simulink subsystem "rss_SensAgCalibNeed"  (R2023a)
settings: Solver=VariableStepAuto  StartTime=0.0  StopTime=10.0  RelTol=1e-3
undefined symbols (not defined in the file): Cdbl_numCalibAlgnNum, Cdbl_trqTqMaxVal, ENM_SYS_STATUS, Gs16_trqRefTqAlgnVal_C, Gu16_ctAlgnAlPhStCnt_C, Gu16_ctAlgnBePhStCnt_C, Gu16_ctAlgnTmpFailStCnt_C, Gu16_ctAlgnWaitAlStCnt_C, Gu16_ctAlgnWaitBeStCnt_C, Gu16_phiAlgnAlPhElecAg_C, Gu16_phiAlgnBePhElecAg_C, Gu16_phiMinAlgnElecAngDvt_C, Gu16_phiTheoBePhElecAg_C
libraries: simulink x1, lib_configurable_parameter x1, vhit_control_library x1, lib_conversion x1
settings Model: Creator=YXQ1WX  LastModifiedBy=xiaoqiang.yuan
settings OptimizationCC: ReuseModelBlockBuffer=off

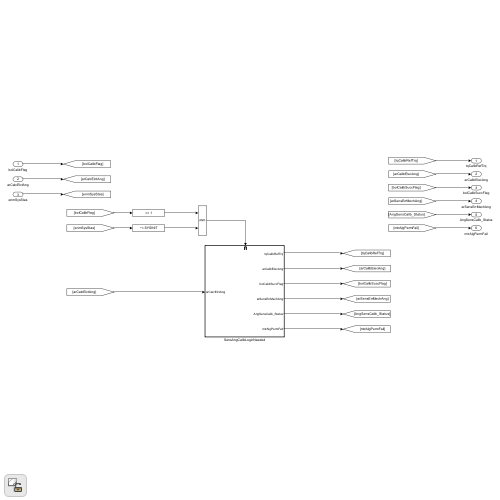
[thumbnail: Simulink's stored preview of the top-level diagram]
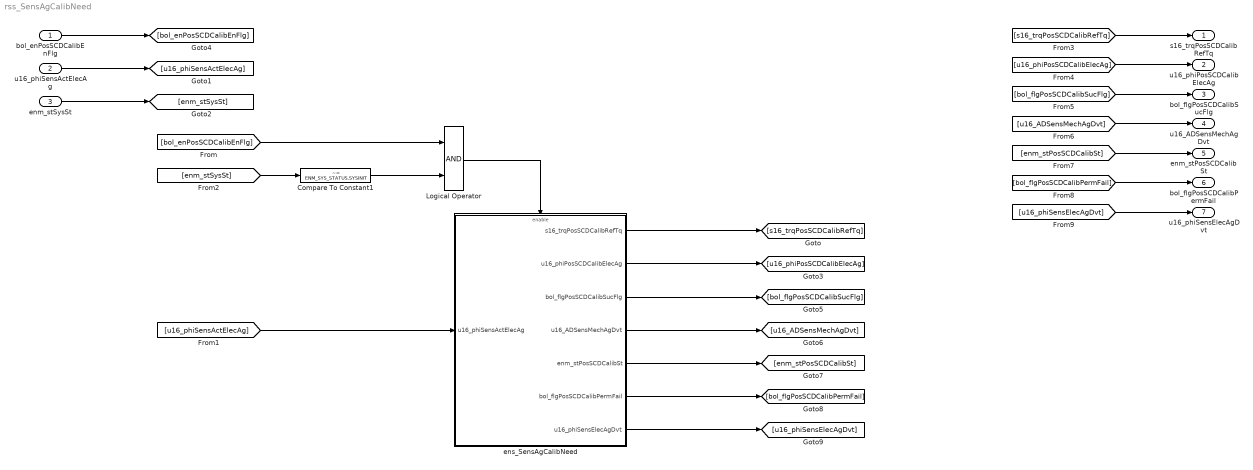
== system rss_SensAgCalibNeed ==
  bol_enPosSCDCalibEnFlg : Inport  OutDataTypeStr=boolean
  u16_phiSensActElecAg : Inport  Port=2  OutDataTypeStr=dt_RadAng_u16r15b0
  enm_stSysSt : Inport  Port=3  OutDataTypeStr=Enum: ENM_SYS_STATUS
  Compare To Constant1 : simulink/Logic and Bit Operations/Compare To Constant  relop=~=  const=ENM_SYS_STATUS.SYSINIT  OutDataTypeStr=boolean
  Logical Operator : Logic  AllPortsSameDT=off  OutDataTypeStr=boolean
  ens_SensAgCalibNeed : Subsystem
  s16_trqPosSCDCalibRefTq : Outport  OutDataTypeStr=dt_Standardize_s16p15b0
  u16_phiPosSCDCalibElecAg : Outport  Port=2  OutDataTypeStr=dt_RadAng_u16r15b0
  bol_flgPosSCDCalibSucFlg : Outport  Port=3  OutDataTypeStr=boolean
  u16_ADSensMechAgDvt : Outport  Port=4  OutDataTypeStr=uint16
  enm_stPosSCDCalibSt : Outport  Port=5  OutDataTypeStr=Enum: ENM_AG_SENS_CALIB_STATUS
  bol_flgPosSCDCalibPermFail : Outport  Port=6  OutDataTypeStr=boolean
  u16_phiSensElecAgDvt : Outport  Port=7  OutDataTypeStr=dt_RadAng_u16r15b0
  wires:
  [u16_phiSensActElecAg] -> ens_SensAgCalibNeed/1(u16_phiSensActElecAg)
  ens_SensAgCalibNeed/1(s16_trqPosSCDCalibRefTq) -> [s16_trqPosSCDCalibRefTq]
  ens_SensAgCalibNeed/2(u16_phiPosSCDCalibElecAg) -> [u16_phiPosSCDCalibElecAg]
  ens_SensAgCalibNeed/3(bol_flgPosSCDCalibSucFlg) -> [bol_flgPosSCDCalibSucFlg]
  ens_SensAgCalibNeed/4(u16_ADSensMechAgDvt) -> [u16_ADSensMechAgDvt]
  ens_SensAgCalibNeed/5(enm_stPosSCDCalibSt) -> [enm_stPosSCDCalibSt]
  ens_SensAgCalibNeed/6(bol_flgPosSCDCalibPermFail) -> [bol_flgPosSCDCalibPermFail]
  Compare To Constant1/1 -> Logical Operator/2
  Logical Operator/1 -> ens_SensAgCalibNeed/Enable
  [bol_enPosSCDCalibEnFlg] -> Logical Operator/1
  [enm_stSysSt] -> Compare To Constant1/1
  bol_enPosSCDCalibEnFlg/1 -> [bol_enPosSCDCalibEnFlg]
  u16_phiSensActElecAg/1 -> [u16_phiSensActElecAg]
  enm_stSysSt/1 -> [enm_stSysSt]
  [s16_trqPosSCDCalibRefTq] -> s16_trqPosSCDCalibRefTq/1
  [u16_phiPosSCDCalibElecAg] -> u16_phiPosSCDCalibElecAg/1
  [bol_flgPosSCDCalibSucFlg] -> bol_flgPosSCDCalibSucFlg/1
  [u16_ADSensMechAgDvt] -> u16_ADSensMechAgDvt/1
  [enm_stPosSCDCalibSt] -> enm_stPosSCDCalibSt/1
  [bol_flgPosSCDCalibPermFail] -> bol_flgPosSCDCalibPermFail/1
  [u16_phiSensElecAgDvt] -> u16_phiSensElecAgDvt/1
  ens_SensAgCalibNeed/7(u16_phiSensElecAgDvt) -> [u16_phiSensElecAgDvt]

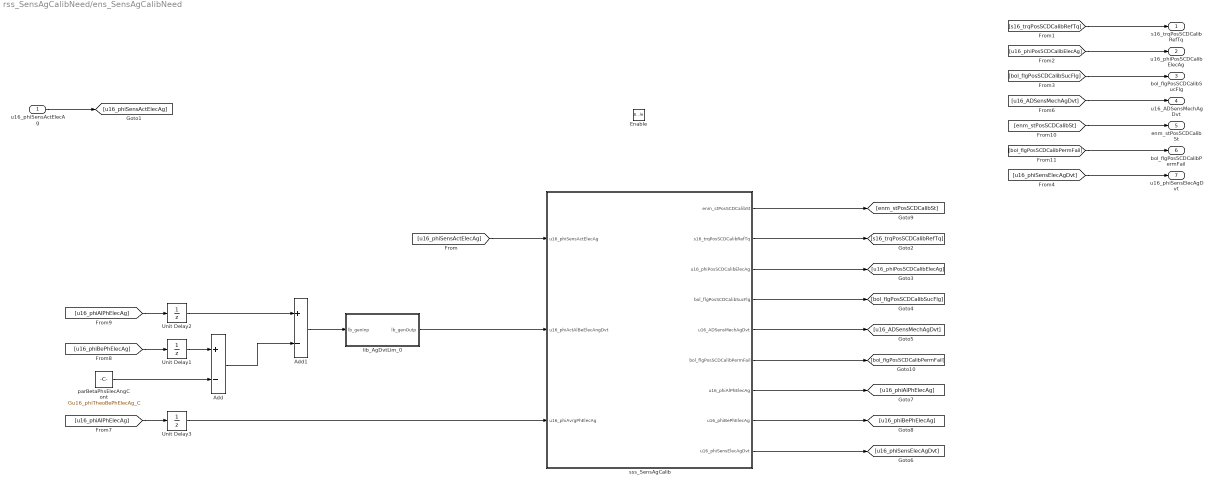
== system rss_SensAgCalibNeed/ens_SensAgCalibNeed ==
  u16_phiSensActElecAg : Inport
  Enable : EnablePort
  Add : Sum  Inputs=+-  RndMeth=Simplest  OutDataTypeStr=Inherit: Same as first input
  Add1 : Sum  Inputs=+-  RndMeth=Simplest  OutDataTypeStr=Inherit: Same as first input
  Unit Delay1 : UnitDelay  SampleTime=-1  HasFrameUpgradeWarning=on
  Unit Delay2 : UnitDelay  SampleTime=-1  HasFrameUpgradeWarning=on
  Unit Delay3 : UnitDelay  SampleTime=-1  HasFrameUpgradeWarning=on
  lib_AgDvtLim_0 : Subsystem
  parBetaPhsElecAngCont : Constant  Value=Gu16_phiTheoBePhElecAg_C
  sss_SensAgCalib : Subsystem
  s16_trqPosSCDCalibRefTq : Outport
  u16_phiPosSCDCalibElecAg : Outport  Port=2
  bol_flgPosSCDCalibSucFlg : Outport  Port=3
  u16_ADSensMechAgDvt : Outport  Port=4
  enm_stPosSCDCalibSt : Outport  Port=5
  bol_flgPosSCDCalibPermFail : Outport  Port=6
  u16_phiSensElecAgDvt : Outport  Port=7
  wires:
  [u16_phiSensElecAgDvt] -> u16_phiSensElecAgDvt/1
  sss_SensAgCalib/9(u16_phiSensElecAgDvt) -> [u16_phiSensElecAgDvt]
  [bol_flgPosSCDCalibPermFail] -> bol_flgPosSCDCalibPermFail/1
  parBetaPhsElecAngCont/1 -> Add/2
  lib_AgDvtLim_0/1(lb_genOutp) -> sss_SensAgCalib/2(u16_phiActAlBeElecAngDvt)
  Add1/1 -> lib_AgDvtLim_0/1(lb_genInp)
  Unit Delay3/1 -> sss_SensAgCalib/3(u16_phiAvrgPhElecAg)
  Unit Delay1/1 -> Add/1
  Add/1 -> Add1/2
  sss_SensAgCalib/6(bol_flgPosSCDCalibPermFail) -> [bol_flgPosSCDCalibPermFail]
  sss_SensAgCalib/3(u16_phiPosSCDCalibElecAg) -> [u16_phiPosSCDCalibElecAg]
  sss_SensAgCalib/5(u16_ADSensMechAgDvt) -> [u16_ADSensMechAgDvt]
  sss_SensAgCalib/7(u16_phiAlPhElecAg) -> [u16_phiAlPhElecAg]
  sss_SensAgCalib/8(u16_phiBePhElecAg) -> [u16_phiBePhElecAg]
  sss_SensAgCalib/4(bol_flgPosSCDCalibSucFlg) -> [bol_flgPosSCDCalibSucFlg]
  [u16_phiAlPhElecAg] -> Unit Delay3/1
  sss_SensAgCalib/2(s16_trqPosSCDCalibRefTq) -> [s16_trqPosSCDCalibRefTq]
  [bol_flgPosSCDCalibSucFlg] -> bol_flgPosSCDCalibSucFlg/1
  [u16_ADSensMechAgDvt] -> u16_ADSensMechAgDvt/1
  [u16_phiSensActElecAg] -> sss_SensAgCalib/1(u16_phiSensActElecAg)
  [s16_trqPosSCDCalibRefTq] -> s16_trqPosSCDCalibRefTq/1
  [u16_phiAlPhElecAg] -> Unit Delay2/1
  [u16_phiPosSCDCalibElecAg] -> u16_phiPosSCDCalibElecAg/1
  Unit Delay2/1 -> Add1/1
  [u16_phiBePhElecAg] -> Unit Delay1/1
  u16_phiSensActElecAg/1 -> [u16_phiSensActElecAg]
  [enm_stPosSCDCalibSt] -> enm_stPosSCDCalibSt/1
  sss_SensAgCalib/1(enm_stPosSCDCalibSt) -> [enm_stPosSCDCalibSt]

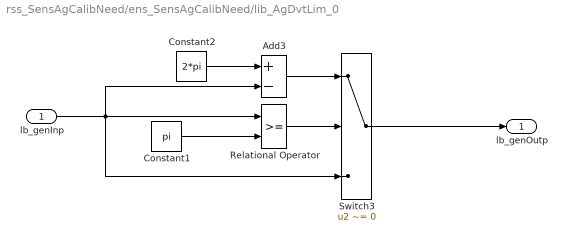
== system rss_SensAgCalibNeed/ens_SensAgCalibNeed/lib_AgDvtLim_0 ==
  lb_genInp : Inport
  Add3 : Sum  Inputs=+-  RndMeth=Simplest  OutDataTypeStr=Inherit: Same as first input
  Constant1 : Constant  Value=pi  OutDataTypeStr=dt_RadAng_u16r15b0
  Constant2 : Constant  Value=2*pi  OutDataTypeStr=dt_RadAng_u16r15b0
  Relational Operator : RelationalOperator  OutDataTypeStr=boolean  RndMeth=Simplest  InputSameDT=off
  Switch3 : Switch  Criteria=u2 ~= 0  RndMeth=Simplest  SaturateOnIntegerOverflow=off  InputSameDT=off  OutDataTypeStr=Inherit: Same as first input
  lb_genOutp : Outport
  wires:
  Relational Operator/1 -> Switch3/2
  Constant2/1 -> Add3/1
  Add3/1 -> Switch3/1
  lb_genInp/1 -> Relational Operator/1, Switch3/3, Add3/2
  Constant1/1 -> Relational Operator/2
  Switch3/1 -> lb_genOutp/1

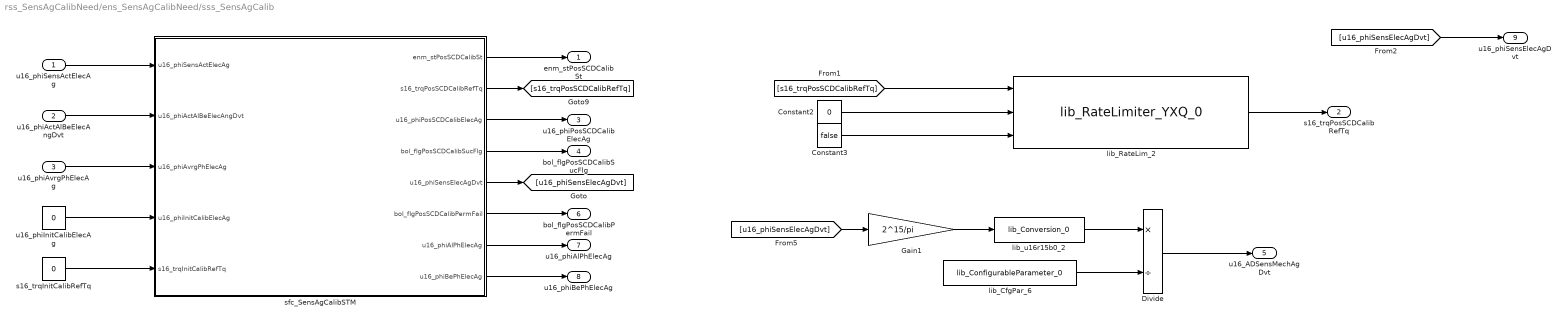
== system rss_SensAgCalibNeed/ens_SensAgCalibNeed/sss_SensAgCalib ==
  u16_phiSensActElecAg : Inport
  u16_phiActAlBeElecAngDvt : Inport  Port=2
  u16_phiAvrgPhElecAg : Inport  Port=3
  Constant2 : Constant  Value=0  OutDataTypeStr=dt_Standardize_s16p15b0
  Constant3 : Constant  Value=false  OutDataTypeStr=boolean
  Divide : Product  Inputs=*/  RndMeth=Simplest  OutDataTypeStr=Inherit: Same as first input
  Gain1 : Gain  Gain=2^15/pi  OutDataTypeStr=Inherit: Inherit via back propagation  RndMeth=Simplest
  lib_CfgPar_6 : lib_configurable_parameter/lib_ConfigurableParameter_0  lb_parCnfgPar=Gu8_numPPNum_C  lb_parDataType=Inherit: Inherit from 'Constant value'  lb_parUpLim=Cdbl_numPPNumMaxVal  lb_parLowLim=Cdbl_numPPNumMinVal
  lib_RateLim_2 : vhit_control_library/lib_RateLimiter_YXQ_0  lb_parSampTime=Cdbl_tiSlwTaskSmpTi  lb_parRiseSlewRate=Gs16_facAlgnTqRiseRate_C  lb_parFallSlewRate=Gs16_facAlgnTqFallRate_C  lb_parMaxInpVal=Cdbl_trqTqMaxVal  lb_parMinInpVal=-Cdbl_trqTqMaxVal
      settings: LibrarySourceBlock=lib_rate_limiter/lib_RateLimiter_0
  lib_u16r15b0_2 : lib_conversion/lib_Conversion_0  lb_parDataType=uint16  lb_parOutpMaxVal=[]  lb_parOutpMinVal=[]  lb_parSatFlag=off
  s16_trqInitCalibRefTq : Constant  Value=0  OutDataTypeStr=dt_Standardize_s16p15b0
  sfc_SensAgCalibSTM : Stateflow chart  TreatAsAtomicUnit=on
  u16_phiInitCalibElecAg : Constant  Value=0  OutDataTypeStr=dt_RadAng_u16r15b0
  enm_stPosSCDCalibSt : Outport
  s16_trqPosSCDCalibRefTq : Outport  Port=2
  u16_phiPosSCDCalibElecAg : Outport  Port=3
  bol_flgPosSCDCalibSucFlg : Outport  Port=4
  u16_ADSensMechAgDvt : Outport  Port=5
  bol_flgPosSCDCalibPermFail : Outport  Port=6
  u16_phiAlPhElecAg : Outport  Port=7
  u16_phiBePhElecAg : Outport  Port=8
  u16_phiSensElecAgDvt : Outport  Port=9
  wires:
  [u16_phiSensElecAgDvt] -> u16_phiSensElecAgDvt/1
  s16_trqInitCalibRefTq/1 -> sfc_SensAgCalibSTM/5(s16_trqInitCalibRefTq)
  u16_phiInitCalibElecAg/1 -> sfc_SensAgCalibSTM/4(u16_phiInitCalibElecAg)
  Constant3/1 -> lib_RateLim_2/3
  [s16_trqPosSCDCalibRefTq] -> lib_RateLim_2/1
  Constant2/1 -> lib_RateLim_2/2
  lib_RateLim_2/1 -> s16_trqPosSCDCalibRefTq/1
  Gain1/1 -> lib_u16r15b0_2/1
  lib_CfgPar_6/1 -> Divide/2
  Divide/1 -> u16_ADSensMechAgDvt/1
  [u16_phiSensElecAgDvt] -> Gain1/1
  lib_u16r15b0_2/1 -> Divide/1
  sfc_SensAgCalibSTM/3(u16_phiPosSCDCalibElecAg) -> u16_phiPosSCDCalibElecAg/1
  sfc_SensAgCalibSTM/2(s16_trqPosSCDCalibRefTq) -> [s16_trqPosSCDCalibRefTq]
  u16_phiActAlBeElecAngDvt/1 -> sfc_SensAgCalibSTM/2(u16_phiActAlBeElecAngDvt)
  u16_phiAvrgPhElecAg/1 -> sfc_SensAgCalibSTM/3(u16_phiAvrgPhElecAg)
  sfc_SensAgCalibSTM/8(u16_phiBePhElecAg) -> u16_phiBePhElecAg/1
  sfc_SensAgCalibSTM/7(u16_phiAlPhElecAg) -> u16_phiAlPhElecAg/1
  sfc_SensAgCalibSTM/5(u16_phiSensElecAgDvt) -> [u16_phiSensElecAgDvt]
  u16_phiSensActElecAg/1 -> sfc_SensAgCalibSTM/1(u16_phiSensActElecAg)
  sfc_SensAgCalibSTM/4(bol_flgPosSCDCalibSucFlg) -> bol_flgPosSCDCalibSucFlg/1
  sfc_SensAgCalibSTM/6(bol_flgPosSCDCalibPermFail) -> bol_flgPosSCDCalibPermFail/1
  sfc_SensAgCalibSTM/1(enm_stPosSCDCalibSt) -> enm_stPosSCDCalibSt/1

== stateflow chart rss_SensAgCalibNeed/ens_SensAgCalibNeed/sss_SensAgCalib/sfc_SensAgCalibSTM ==
  state ALIGN_ALPHA_PHASE1
    en:
    enm_stPosSCDCalibSt = ENM_AG_SENS_CALIB_STATUS.ALPHA_PHASE1;
    s16_trqPosSCDCalibRefTq = Gs16_trqRefTqAlgnVal_C;
    u16_phiPosSCDCalibElecAg = Gu16_phiAlgnAlPhElecAg_C;
    bol_flgPosSCDCalibSucFlg = false;
    bol_flgPosSCDCalibPermFail = false;
    u16_ctCalibStWaitCnt = uint16(0);
    du:
    u16_ctCalibStWaitCnt = u16_ctCalibStWaitCnt + uint16(1);
    ex:
    u16_ctCalibStWaitCnt = uint16(0);
    u16_phiAlPhElecAg = u16_phiSensActElecAg;
  state WAIT_ALPHA1
    en:
    enm_stPosSCDCalibSt = ENM_AG_SENS_CALIB_STATUS.WAIT_ALPHA1;
    s16_trqPosSCDCalibRefTq =s16_trqInitCalibRefTq;
    u16_phiPosSCDCalibElecAg = u16_phiInitCalibElecAg;
    bol_flgPosSCDCalibSucFlg = false;
    bol_flgPosSCDCalibPermFail = false;
    u16_ctCalibStWaitCnt = uint16(0);
    du:
    u16_ctCalibStWaitCnt = u16_ctCalibStWaitCnt + uint16(1);
    ex:
    u16_ctCalibStWaitCnt = uint16(0);
  state ALIGN_BETA_PHASE
    en:
    enm_stPosSCDCalibSt = ENM_AG_SENS_CALIB_STATUS.BETA_PHASE;
    s16_trqPosSCDCalibRefTq = Gs16_trqRefTqAlgnVal_C;
    u16_phiPosSCDCalibElecAg = Gu16_phiAlgnBePhElecAg_C;
    bol_flgPosSCDCalibSucFlg = false;
    bol_flgPosSCDCalibPermFail = false;
    u16_ctCalibStWaitCnt = uint16(0);
    du:
    u16_ctCalibStWaitCnt = u16_ctCalibStWaitCnt + uint16(1);
    ex:
    u16_ctCalibStWaitCnt = uint16(0);
    u16_phiBePhElecAg = u16_phiSensActElecAg;
  state WAIT_BETA
    en:
    enm_stPosSCDCalibSt = ENM_AG_SENS_CALIB_STATUS.WAIT_BETA;
    s16_trqPosSCDCalibRefTq = s16_trqInitCalibRefTq;
    u16_phiPosSCDCalibElecAg = u16_phiInitCalibElecAg;
    bol_flgPosSCDCalibSucFlg = false;
    bol_flgPosSCDCalibPermFail = false;
    u16_ctCalibStWaitCnt = uint16(0);
    du:
    u16_ctCalibStWaitCnt = u16_ctCalibStWaitCnt + uint16(1);
    ex:
    u16_ctCalibStWaitCnt = uint16(0);
    u8_ctTryAlgCnt = u8_ctTryAlgCnt + uint8(1);
  state ALIGN_ALPHA_PHASE2
    en:
    enm_stPosSCDCalibSt = ENM_AG_SENS_CALIB_STATUS.ALPHA_PHASE2;
    s16_trqPosSCDCalibRefTq = Gs16_trqRefTqAlgnVal_C;
    u16_phiPosSCDCalibElecAg = Gu16_phiAlgnAlPhElecAg_C;
    bol_flgPosSCDCalibSucFlg = false;
    bol_flgPosSCDCalibPermFail = false;
    u16_ctCalibStWaitCnt = uint16(0);
    du:
    u16_ctCalibStWaitCnt = u16_ctCalibStWaitCnt + uint16(1);
    ex:
    u16_ctCalibStWaitCnt = uint16(0);
    u16_phiAlPhElecAg = u16_phiSensActElecAg;
  state CALIBFAIL
    en:
    enm_stPosSCDCalibSt = ENM_AG_SENS_CALIB_STATUS.CALIBFAIL;
    s16_trqPosSCDCalibRefTq = s16_trqInitCalibRefTq;
    u16_phiPosSCDCalibElecAg = u16_phiInitCalibElecAg;
    bol_flgPosSCDCalibSucFlg = false;
    if (u8_ctTryAlgCnt == uint8(Cdbl_numCalibAlgnNum));
    bol_flgPosSCDCalibPermFail = true;
    end;
    u16_ctCalibStWaitCnt = uint16(0);
    du:
    if (u8_ctTryAlgCnt < uint8(Cdbl_numCalibAlgnNum));
    u16_ctCalibStWaitCnt = u16_ctCalibStWaitCnt + uint16(1);
    else;
    u16_ctCalibStWaitCnt = uint16(0);
    end;
    ex:
    u16_ctCalibStWaitCnt = uint16(0);
  state WAIT_ALPHA2
    en:
    enm_stPosSCDCalibSt = ENM_AG_SENS_CALIB_STATUS.WAIT_ALPHA2;
    s16_trqPosSCDCalibRefTq =s16_trqInitCalibRefTq;
    u16_phiPosSCDCalibElecAg = u16_phiInitCalibElecAg;
    bol_flgPosSCDCalibSucFlg = false;
    bol_flgPosSCDCalibPermFail = false;
    u16_ctCalibStWaitCnt = uint16(0);
    du:
    u16_ctCalibStWaitCnt = u16_ctCalibStWaitCnt + uint16(1);
    ex:
    u16_ctCalibStWaitCnt = uint16(0);
  state SUCCESS
    en:
    enm_stPosSCDCalibSt = ENM_AG_SENS_CALIB_STATUS.SUCCESS;
    s16_trqPosSCDCalibRefTq = s16_trqInitCalibRefTq;
    u16_phiPosSCDCalibElecAg = u16_phiInitCalibElecAg;
    bol_flgPosSCDCalibSucFlg = true;
    u16_phiSensElecAgDvt = u16_phiAvrgPhElecAg;
    bol_flgPosSCDCalibPermFail = false;
  (default) -> ALIGN_ALPHA_PHASE1 : {u16_ctCalibStWaitCnt = uint16(0);
      | u8_ctTryAlgCnt = uint8(0);}
  ALIGN_ALPHA_PHASE1 -> WAIT_ALPHA1 : [u16_ctCalibStWaitCnt >= Gu16_ctAlgnAlPhStCnt_C]
  WAIT_ALPHA1 -> ALIGN_BETA_PHASE : [u16_ctCalibStWaitCnt >= Gu16_ctAlgnWaitAlStCnt_C]
  CALIBFAIL -> ALIGN_ALPHA_PHASE1 : [u16_ctCalibStWaitCnt >= Gu16_ctAlgnTmpFailStCnt_C]
  ALIGN_BETA_PHASE -> WAIT_BETA : [u16_ctCalibStWaitCnt >= Gu16_ctAlgnBePhStCnt_C]
  WAIT_BETA -> ALIGN_ALPHA_PHASE2 : [u16_ctCalibStWaitCnt >= Gu16_ctAlgnWaitBeStCnt_C]
  ALIGN_ALPHA_PHASE2 -> WAIT_ALPHA2 : [u16_ctCalibStWaitCnt >= Gu16_ctAlgnAlPhStCnt_C]
  WAIT_ALPHA2 -> SUCCESS [order 1] : [u16_ctCalibStWaitCnt >= Gu16_ctAlgnWaitAlStCnt_C && ...
      | u16_phiActAlBeElecAngDvt <= Gu16_phiMinAlgnElecAngDvt_C]
  WAIT_ALPHA2 -> CALIBFAIL [order 2] : [u16_ctCalibStWaitCnt >= Gu16_ctAlgnWaitAlStCnt_C && ...
      | u16_phiActAlBeElecAngDvt > Gu16_phiMinAlgnElecAngDvt_C]
  data: Gu16_ctAlgnAlPhStCnt_C parameter; Gu16_ctAlgnBePhStCnt_C parameter; u8_ctTryAlgCnt local uint8; Cdbl_numCalibAlgnNum parameter; Gs16_trqRefTqAlgnVal_C parameter; Gu16_phiAlgnAlPhElecAg_C parameter; u16_ctCalibStWaitCnt local uint16; Gu16_phiAlgnBePhElecAg_C parameter; Gu16_phiMinAlgnElecAngDvt_C parameter; enm_stPosSCDCalibSt output Enum: ENM_AG_SENS_CALIB_STATUS; s16_trqPosSCDCalibRefTq output dt_Standardize_s16p15b0; u16_phiPosSCDCalibElecAg output dt_RadAng_u16r15b0; bol_flgPosSCDCalibSucFlg output boolean; u16_phiSensElecAgDvt output dt_RadAng_u16r15b0; bol_flgPosSCDCalibPermFail output boolean; u16_phiSensActElecAg input dt_RadAng_u16r15b0; Gu16_ctAlgnTmpFailStCnt_C parameter; u16_phiAlPhElecAg output dt_RadAng_u16r15b0; u16_phiBePhElecAg output dt_RadAng_u16r15b0; u16_phiActAlBeElecAngDvt input dt_RadAng_u16r15b0; u16_phiAvrgPhElecAg input dt_RadAng_u16r15b0; Gu16_ctAlgnWaitAlStCnt_C parameter; Gu16_ctAlgnWaitBeStCnt_C parameter; u16_phiInitCalibElecAg input dt_RadAng_u16r15b0; s16_trqInitCalibRefTq input dt_Standardize_s16p15b0
